simulink model "untitled"  (R2016b)
settings: Solver=VariableStepAuto  StartTime=0.0  StopTime=inf  RelTol=1e-3
undefined symbols (not defined in the file): serial
libraries: instrumentlib x2
settings Model: Creator=ricky  LastModifiedBy=ricky

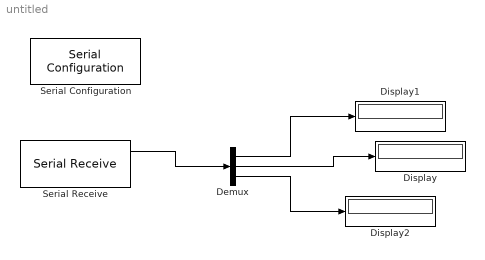
== system untitled ==
  Demux : Demux  Outputs=3
  Display : Display
  Display1 : Display
  Display2 : Display
  Serial Configuration : instrumentlib/Serial Configuration  Priority=-200000  ComPortMenu=<Please select a port...>  ComPort=COM11  ObjConstructor=serial('COM11');  BaudRate=57600  DataBits=8  Parity=none  FlowControl=none  Timeout=10  ByteOrder=LittleEndian
  Serial Receive : instrumentlib/Serial Receive  ComPortMenu=COM11  ComPort=COM11  ObjConstructor=serial('COM11');  Terminator=<none>  DataSize="[3  1]"  DataType=single  EnableBlockingMode=off  ActionDataUnavailable=Output last received value  CustomValue=0  SampleTime=0.01
  wires:
  Serial Receive/1 -> Demux/1
  Demux/1 -> Display1/1
  Demux/2 -> Display/1
  Demux/3 -> Display2/1
